simulink model "PlantIdentification"  (R2025b)
settings: Solver=VariableStepAuto  StartTime=0.0  StopTime=20  RelTol=1e-3
values from neighbouring files (symbols this model uses):
  Ts_meas = 0.005    [ctrlSys.sldd]
libraries: commseqgen3 x1, simulink x1
settings Model: DataDictionary=ctrlSys.sldd  SimulationMode=accelerator  Creator=LYG  LastModifiedBy=A

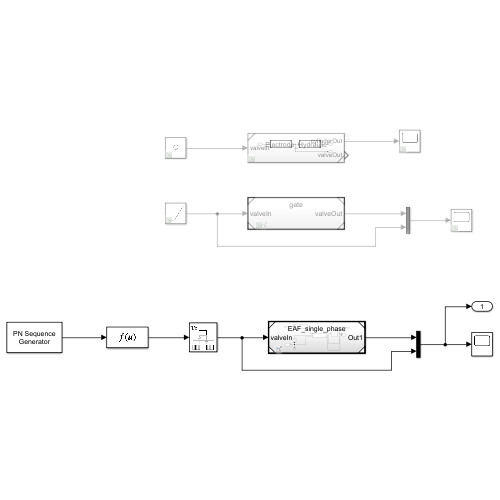
[thumbnail: Simulink's stored preview of the top-level diagram]
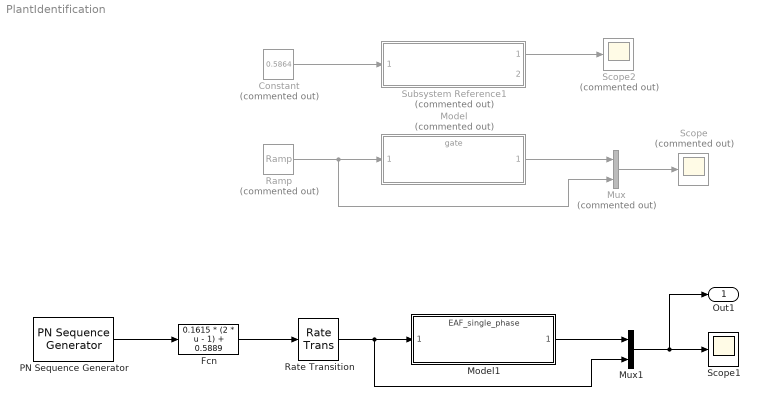
== system PlantIdentification ==
  Constant : Constant  Commented=on  Value=0.5864
  Fcn : Fcn  Expr=0.1615 * (2 * u - 1) + 0.5889
  Model : ModelReference  Commented=on  ModelNameDialog=gate.slx  SimulationMode=Normal  ModelReferenceVersion=3.11
  Model1 : ModelReference  ModelNameDialog=EAF_single_phase.slx  SimulationMode=Normal  ModelReferenceVersion=1.16
  Mux : Mux  Commented=on  Inputs=2
  Mux1 : Mux  Inputs=2
  PN Sequence Generator : commseqgen3/PN Sequence Generator  poly='z^6 + z + 1'  ini_sta=[0 0 0 0 0 1]  outBitMaskSource=Dialog parameter  shift=0  outVarSiz=off  maxOutSizeMode=Dialog parameter  maxOutSize=[10 1]  Ts=Ts_meas  sampPerFrame=sample_per_frame  reset=off  bitPackedOutputs=off  outDataType=double  numPackedBits=8  bitPackDataSigned=off  bitPackedOutDType=double
      settings: LibrarySourceBlock=|
      | commhdlsource/PN Sequence
      | Generator
  Ramp : simulink/Sources/Ramp  Commented=on  slope=0.4  start=0  InitialOutput=-2
  Rate Transition : RateTransition  InitialCondition=0.6  OutPortSampleTime=Ts_local
  Scope : Scope  Commented=on
      settings: ActiveDisplayYMinimum=-0.00525  ActiveDisplayYMaximum=0.0072499999999999995
  Scope1 : Scope
      settings: ActiveDisplayYMinimum=-0.0050445162376974431  ActiveDisplayYMaximum=0.045400646139276996
  Scope2 : Scope  Commented=on
      settings: ActiveDisplayYMinimum=-0.00525  ActiveDisplayYMaximum=0.0072499999999999995  DataLoggingVariableName=ScopeData2
  Subsystem Reference1 : Subsystem  Commented=on  ReferencedSubsystem=Electrode_Hydraulic
  Out1 : Outport
  wires:
  Ramp/1 -> Mux/2, Model/1
  Model/1 -> Mux/1
  Mux/1 -> Scope/1
  PN Sequence Generator/1 -> Fcn/1
  Model1/1 -> Mux1/1
  Mux1/1 -> Out1/1, Scope1/1
  Fcn/1 -> Rate Transition/1
  Rate Transition/1 -> Mux1/2, Model1/1
  Constant/1 -> Subsystem Reference1/1
  Subsystem Reference1/1 -> Scope2/1
